simulink model "GCI_Ctrl_PLL_C2000"  (R2024a)
settings: Solver=FixedStepDiscrete  StartTime=0.0  StopTime=8  FixedStep=Sim.ContSampleTime  RelTol=1e-3  EnableMultiTasking=on
values from neighbouring files (symbols this model uses):
  ADPTV = 1.3912    [ModelDD.sldd]
  Ctrl = 0    [ModelDD.sldd]
  EnableMonitors = 0    [ModelDD.sldd]
  FrcPwr = 1    [ModelDD.sldd]
  IdSp = 0.0    [ModelDD.sldd]
  IqSp = 0.0    [ModelDD.sldd]
  ModReq = 1    [ModelDD.sldd]
  PorISel = 0    [ModelDD.sldd]
  PSp = 0.0    [ModelDD.sldd]
  QSp = 0.0    [ModelDD.sldd]
  Sim : value not decoded    [ModelDD.sldd]
  Test = 0    [ModelDD.sldd]
  Var = 650.0    [ModelDD.sldd]
undefined symbols (not defined in the file or in its folder): DiscIntNeverNeededParam, Down, GPTRIP1SEL, GPTRIP2SEL, magnitude, P, TZ1, TZ2, Up
libraries: simulink x38, c2837xDlib x22, c2802xlib x15, slpidlib x9, spsMeanLib x9, spsCurrentMeasurementLib x7, spsThreePhaseVIMeasurementLib x5, spsVoltageMeasurementLib x5, spsTHDLib x4, spsSeriesRLCBranchLib x4, svdutilitieslib x3, c280xlib x3
(part 11 of 11)

== system GCI_Ctrl_PLL_C2000/C2000_SW/CtrlLoop/CurrentController/FeedForward/Subsystem/abc_dqz/Subsystem2 ==
  note: [  al
      |     be  ]
  note: q = -al*sin(wt) + be*cos(wt)
  note: [  cos(wt)   sin(wt)
      |    -sin(wt)    cos(wt)   ]
  note: d = al*cos(wt) + be*sin(wt)
  note: [ d
      |    q ]
  note: *
  note: =
  alpha_beta : Inport
  Ang : Inport  Port=2  PortDimensions=1
  Fcn : Fcn  Expr=u[1]*cos(u[3]) + u[2]*sin(u[3])
  Fcn1 : Fcn  Expr=-u[1]*sin(u[3]) + u[2]*cos(u[3])
  Mux : Mux  Inputs=3
  Mux1 : Mux  Inputs=[2 1]
  Mux2 : Mux  Inputs=[2 1]
  Selector : Selector  InputPortWidth=3  IndexOptions=Index vector (dialog)  Indices=[1 2]  OutputSizes=1
  Selector1 : Selector  InputPortWidth=3  IndexOptions=Index vector (dialog)  Indices=[3]  OutputSizes=1
  dq : Outport  InitialOutput=[0,0]  VectorParamsAs1DForOutWhenUnconnected=off
  wires:
  Selector1/1 -> Mux/3
  Selector/1 -> Mux1/1, Mux2/1
  Mux2/1 -> Fcn1/1
  Mux/1 -> dq/1
  Ang/1 -> Mux1/2, Mux2/2
  Fcn/1 -> Mux/1
  Fcn1/1 -> Mux/2
  Mux1/1 -> Fcn/1
  alpha_beta/1 -> Selector1/1, Selector/1

== system GCI_Ctrl_PLL_C2000/C2000_SW/CtrlLoop/CurrentController/FeedForward/Subsystem/dd_dqz1/LPF ==
  u : Inport
  Alpha : Gain  Gain=(2-w*Ts)/(2+w*Ts)
  Beta : Gain  Gain=(w*Ts)/(2+w*Ts)
  Delay1 : Delay  DelayLength=1  InitialCondition=y_0
  Delay2 : Delay  DelayLength=1
  Sum1 : Sum  Inputs=++|
  Sum2 : Sum  Inputs=|++
  y : Outport  VectorParamsAs1DForOutWhenUnconnected=off
  wires:
  u/1 -> Sum1/1, Delay2/1
  Delay1/1 -> Alpha/1  "y(n-1)"
  Alpha/1 -> Sum2/2
  Delay2/1 -> Sum1/2
  Sum1/1 -> Beta/1
  Beta/1 -> Sum2/1
  Sum2/1 -> Delay1/1, y/1

== system GCI_Ctrl_PLL_C2000/C2000_SW/CtrlLoop/CurrentController/FeedForward/Subsystem/dd_dqz1/LPF1 ==
  u : Inport
  Alpha : Gain  Gain=(2-w*Ts)/(2+w*Ts)
  Beta : Gain  Gain=(w*Ts)/(2+w*Ts)
  Delay1 : Delay  DelayLength=1  InitialCondition=y_0
  Delay2 : Delay  DelayLength=1
  Sum1 : Sum  Inputs=++|
  Sum2 : Sum  Inputs=|++
  y : Outport  VectorParamsAs1DForOutWhenUnconnected=off
  wires:
  Sum2/1 -> y/1, Delay1/1
  Beta/1 -> Sum2/1
  Sum1/1 -> Beta/1
  Delay2/1 -> Sum1/2
  Alpha/1 -> Sum2/2
  Delay1/1 -> Alpha/1  "y(n-1)"
  u/1 -> Delay2/1, Sum1/1

== system GCI_Ctrl_PLL_C2000/C2000_SW/CtrlLoop/CurrentController/FeedForward/Subsystem/dd_dqz1/Subsystem ==
  abc : Inport  PortDimensions=3
  Gain1 : Gain  Gain=single(2/3)  ParamDataTypeStr=single  SaturateOnIntegerOverflow=on  OutDataTypeStr=Inherit: Same as input
  Gain3 : Gain  Gain="single([ 1   -1/2   -1/2; 0   sqrt(3)/2   -sqrt(3)/2; 1/2  1/2  1/2 ] )"  Multiplication=Matrix(K*u) (u vector)  ParamDataTypeStr=single  SaturateOnIntegerOverflow=on  OutDataTypeStr=Inherit: Same as input
  al_be_0 : Outport  VectorParamsAs1DForOutWhenUnconnected=off
  wires:
  abc/1 -> Gain3/1
  Gain3/1 -> Gain1/1
  Gain1/1 -> al_be_0/1  "AlphaBetaZero"

== system GCI_Ctrl_PLL_C2000/C2000_SW/CtrlLoop/CurrentController/FeedForward/Subsystem/dd_dqz1/Subsystem1 ==
  note: =
  note: *
  note: [ d
      |    q ]
  note: d = al*cos(wt) + be*sin(wt)
  note: [  cos(wt)   sin(wt)
      |    -sin(wt)    cos(wt)   ]
  note: q = -al*sin(wt) + be*cos(wt)
  note: [  al
      |     be  ]
  alpha_beta : Inport
  wtNow : Inport  Port=2  PortDimensions=1
  Fcn : Fcn  Expr=u[1]*cos(u[3]) + u[2]*sin(u[3])
  Fcn1 : Fcn  Expr=-u[1]*sin(u[3]) + u[2]*cos(u[3])
  Mux : Mux  Inputs=3
  Mux1 : Mux  Inputs=[2 1]
  Mux2 : Mux  Inputs=[2 1]
  Selector : Selector  InputPortWidth=3  IndexOptions=Index vector (dialog)  Indices=[1 2]  OutputSizes=1
  Selector1 : Selector  InputPortWidth=3  IndexOptions=Index vector (dialog)  Indices=[3]  OutputSizes=1
  dq : Outport  InitialOutput=[0,0]  VectorParamsAs1DForOutWhenUnconnected=off
  wires:
  alpha_beta/1 -> Selector/1, Selector1/1
  Mux1/1 -> Fcn/1
  Fcn1/1 -> Mux/2
  Fcn/1 -> Mux/1
  wtNow/1 -> Mux2/2, Mux1/2
  Mux/1 -> dq/1
  Mux2/1 -> Fcn1/1
  Selector/1 -> Mux2/1, Mux1/1
  Selector1/1 -> Mux/3

== system GCI_Ctrl_PLL_C2000/C2000_SW/CtrlLoop/CurrentController/FeedForward/Subsystem/dd_dqz1/Subsystem2 ==
  note: [  al
      |     be  ]
  note: q = -al*sin(wt) + be*cos(wt)
  note: [  cos(wt)   sin(wt)
      |    -sin(wt)    cos(wt)   ]
  note: d = al*cos(wt) + be*sin(wt)
  note: [ d
      |    q ]
  note: *
  note: =
  alpha_beta : Inport
  wtNow : Inport  Port=2  PortDimensions=1
  Fcn : Fcn  Expr=u[1]*cos(u[3]) + u[2]*sin(u[3])
  Fcn1 : Fcn  Expr=-u[1]*sin(u[3]) + u[2]*cos(u[3])
  Mux : Mux  Inputs=3
  Mux1 : Mux  Inputs=[2 1]
  Mux2 : Mux  Inputs=[2 1]
  Selector : Selector  InputPortWidth=3  IndexOptions=Index vector (dialog)  Indices=[1 2]  OutputSizes=1
  Selector1 : Selector  InputPortWidth=3  IndexOptions=Index vector (dialog)  Indices=[3]  OutputSizes=1
  dq : Outport  InitialOutput=[0,0]  VectorParamsAs1DForOutWhenUnconnected=off
  wires:
  Selector1/1 -> Mux/3
  Selector/1 -> Mux1/1, Mux2/1
  Mux2/1 -> Fcn1/1
  Mux/1 -> dq/1
  Fcn/1 -> Mux/1
  Fcn1/1 -> Mux/2
  Mux1/1 -> Fcn/1
  alpha_beta/1 -> Selector1/1, Selector/1
  wtNow/1 -> Mux2/2, Mux1/2

== system GCI_Ctrl_PLL_C2000/C2000_SW/CtrlLoop/CurrentController/FeedForward/Subsystem/dd_dqz1/Subsystem3 ==
  Vdq_in : Inport
  Vdq_Inverse : Inport  Port=2
  Theta : Inport  Port=3
  Cos : Trigonometry  Operator=cos
  Demux1 : Demux  Outputs=2
  Demux2 : Demux  Outputs=2
  Gain : Gain  Gain=2  ParamDataTypeStr=single
  Ground : Ground
  Mux : Mux  Inputs=3
  Product{,1..3} (4 alike) : Product
  Selector : Selector  InputPortWidth=3  IndexOptions=Index vector (dialog)  Indices=[1 2]  OutputSizes=1
  Selector1 : Selector  InputPortWidth=3  IndexOptions=Index vector (dialog)  Indices=[1 2]  OutputSizes=1
  Sin : Trigonometry
  Sum : Sum  Inputs=|+-
  Sum1 : Sum  Inputs=|++
  Sum2 : Sum  Inputs=|+-
  Sum3 : Sum  Inputs=|+-
  Vdq_out : Outport  VectorParamsAs1DForOutWhenUnconnected=off
  wires:
  Ground/1 -> Mux/3
  Mux/1 -> Vdq_out/1
  Sum3/1 -> Mux/2
  Product3/1 -> Sum3/2
  Sum1/1 -> Sum3/1
  [Vq_Neg] -> Product3/1
  [Cos] -> Product3/2
  Product2/1 -> Sum2/2
  [Vq_Neg] -> Product2/1
  [Sin] -> Product2/2
  Sum2/1 -> Mux/1
  Sum/1 -> Sum2/1
  [Vq_Pos] -> Sum1/1
  Product1/1 -> Sum1/2
  [Vd_Neg] -> Product1/1
  [Sin] -> Product1/2
  [Cos] -> Product/2
  [Vd_Neg] -> Product/1
  Product/1 -> Sum/2
  Cos/1 -> [Cos]
  Sin/1 -> [Sin]
  [Vd_Pos] -> Sum/1
  Demux1/2 -> [Vq_Neg]
  Demux1/1 -> [Vd_Neg]
  Demux2/2 -> [Vq_Pos]
  Demux2/1 -> [Vd_Pos]
  Vdq_Inverse/1 -> Selector1/1
  Selector1/1 -> Demux1/1
  Selector/1 -> Demux2/1
  Vdq_in/1 -> Selector/1
  Gain/1 -> Sin/1, Cos/1
  Theta/1 -> Gain/1

== system GCI_Ctrl_PLL_C2000/C2000_SW/CtrlLoop/CurrentController/FeedForward/Subsystem/dd_dqz1/Subsystem4 ==
  Vdq_in : Inport
  Vdq_Inverse : Inport  Port=2
  Theta : Inport  Port=3
  Cos : Trigonometry  Operator=cos
  Demux1 : Demux  Outputs=2
  Demux2 : Demux  Outputs=2
  Gain : Gain  Gain=2  ParamDataTypeStr=single
  Ground : Ground
  Mux : Mux  Inputs=3
  Product{,1..3} (4 alike) : Product
  Selector : Selector  InputPortWidth=3  IndexOptions=Index vector (dialog)  Indices=[1 2]  OutputSizes=1
  Selector1 : Selector  InputPortWidth=3  IndexOptions=Index vector (dialog)  Indices=[1 2]  OutputSizes=1
  Sin : Trigonometry
  Sum : Sum  Inputs=|+-
  Sum1 : Sum  Inputs=|++
  Sum2 : Sum  Inputs=|+-
  Sum3 : Sum  Inputs=|+-
  Vdq_out : Outport  VectorParamsAs1DForOutWhenUnconnected=off
  wires:
  Theta/1 -> Gain/1
  Gain/1 -> Cos/1, Sin/1
  Vdq_in/1 -> Selector/1
  Selector/1 -> Demux2/1
  Selector1/1 -> Demux1/1
  Vdq_Inverse/1 -> Selector1/1
  Demux2/1 -> [Vd_Pos]
  Demux2/2 -> [Vq_Pos]
  Demux1/1 -> [Vd_Neg]
  Demux1/2 -> [Vq_Neg]
  [Vd_Pos] -> Sum/1
  Sin/1 -> [Sin]
  Cos/1 -> [Cos]
  Product/1 -> Sum/2
  [Vd_Neg] -> Product/1
  [Cos] -> Product/2
  [Sin] -> Product1/2
  [Vd_Neg] -> Product1/1
  Product1/1 -> Sum1/2
  [Vq_Pos] -> Sum1/1
  Sum/1 -> Sum2/1
  Sum2/1 -> Mux/1
  [Sin] -> Product2/2
  [Vq_Neg] -> Product2/1
  Product2/1 -> Sum2/2
  [Cos] -> Product3/2
  [Vq_Neg] -> Product3/1
  Sum1/1 -> Sum3/1
  Product3/1 -> Sum3/2
  Sum3/1 -> Mux/2
  Mux/1 -> Vdq_out/1
  Ground/1 -> Mux/3

== system GCI_Ctrl_PLL_C2000/C2000_SW/CtrlLoop/CurrentController/FeedForward/Subsystem/dd_dqz2/LPF ==
  u : Inport
  Alpha : Gain  Gain=(2-w*Ts)/(2+w*Ts)
  Beta : Gain  Gain=(w*Ts)/(2+w*Ts)
  Delay1 : Delay  DelayLength=1  InitialCondition=y_0
  Delay2 : Delay  DelayLength=1
  Sum1 : Sum  Inputs=++|
  Sum2 : Sum  Inputs=|++
  y : Outport  VectorParamsAs1DForOutWhenUnconnected=off
  wires:
  u/1 -> Sum1/1, Delay2/1
  Delay1/1 -> Alpha/1  "y(n-1)"
  Alpha/1 -> Sum2/2
  Delay2/1 -> Sum1/2
  Sum1/1 -> Beta/1
  Beta/1 -> Sum2/1
  Sum2/1 -> Delay1/1, y/1

== system GCI_Ctrl_PLL_C2000/C2000_SW/CtrlLoop/CurrentController/FeedForward/Subsystem/dd_dqz2/LPF1 ==
  u : Inport
  Alpha : Gain  Gain=(2-w*Ts)/(2+w*Ts)
  Beta : Gain  Gain=(w*Ts)/(2+w*Ts)
  Delay1 : Delay  DelayLength=1  InitialCondition=y_0
  Delay2 : Delay  DelayLength=1
  Sum1 : Sum  Inputs=++|
  Sum2 : Sum  Inputs=|++
  y : Outport  VectorParamsAs1DForOutWhenUnconnected=off
  wires:
  Sum2/1 -> y/1, Delay1/1
  Beta/1 -> Sum2/1
  Sum1/1 -> Beta/1
  Delay2/1 -> Sum1/2
  Alpha/1 -> Sum2/2
  Delay1/1 -> Alpha/1  "y(n-1)"
  u/1 -> Delay2/1, Sum1/1

== system GCI_Ctrl_PLL_C2000/C2000_SW/CtrlLoop/CurrentController/FeedForward/Subsystem/dd_dqz2/Subsystem ==
  abc : Inport  PortDimensions=3
  Gain1 : Gain  Gain=single(2/3)  ParamDataTypeStr=single  SaturateOnIntegerOverflow=on  OutDataTypeStr=Inherit: Same as input
  Gain3 : Gain  Gain="single([ 1   -1/2   -1/2; 0   sqrt(3)/2   -sqrt(3)/2; 1/2  1/2  1/2 ] )"  Multiplication=Matrix(K*u) (u vector)  ParamDataTypeStr=single  SaturateOnIntegerOverflow=on  OutDataTypeStr=Inherit: Same as input
  al_be_0 : Outport  VectorParamsAs1DForOutWhenUnconnected=off
  wires:
  Gain1/1 -> al_be_0/1  "AlphaBetaZero"
  Gain3/1 -> Gain1/1
  abc/1 -> Gain3/1

== system GCI_Ctrl_PLL_C2000/C2000_SW/CtrlLoop/CurrentController/FeedForward/Subsystem/dd_dqz2/Subsystem1 ==
  note: [  al
      |     be  ]
  note: q = -al*sin(wt) + be*cos(wt)
  note: [  cos(wt)   sin(wt)
      |    -sin(wt)    cos(wt)   ]
  note: d = al*cos(wt) + be*sin(wt)
  note: [ d
      |    q ]
  note: *
  note: =
  alpha_beta : Inport
  wtNow : Inport  Port=2  PortDimensions=1
  Fcn : Fcn  Expr=u[1]*cos(u[3]) + u[2]*sin(u[3])
  Fcn1 : Fcn  Expr=-u[1]*sin(u[3]) + u[2]*cos(u[3])
  Mux : Mux  Inputs=3
  Mux1 : Mux  Inputs=[2 1]
  Mux2 : Mux  Inputs=[2 1]
  Selector : Selector  InputPortWidth=3  IndexOptions=Index vector (dialog)  Indices=[1 2]  OutputSizes=1
  Selector1 : Selector  InputPortWidth=3  IndexOptions=Index vector (dialog)  Indices=[3]  OutputSizes=1
  dq : Outport  InitialOutput=[0,0]  VectorParamsAs1DForOutWhenUnconnected=off
  wires:
  Selector1/1 -> Mux/3
  Selector/1 -> Mux1/1, Mux2/1
  Mux2/1 -> Fcn1/1
  Mux/1 -> dq/1  "dq"
  wtNow/1 -> Mux1/2, Mux2/2
  Fcn/1 -> Mux/1
  Fcn1/1 -> Mux/2
  Mux1/1 -> Fcn/1
  alpha_beta/1 -> Selector1/1, Selector/1

== system GCI_Ctrl_PLL_C2000/C2000_SW/CtrlLoop/CurrentController/FeedForward/Subsystem/dd_dqz2/Subsystem2 ==
  note: =
  note: *
  note: [ d
      |    q ]
  note: d = al*cos(wt) + be*sin(wt)
  note: [  cos(wt)   sin(wt)
      |    -sin(wt)    cos(wt)   ]
  note: q = -al*sin(wt) + be*cos(wt)
  note: [  al
      |     be  ]
  alpha_beta : Inport
  wtNow : Inport  Port=2  PortDimensions=1
  Fcn : Fcn  Expr=u[1]*cos(u[3]) + u[2]*sin(u[3])
  Fcn1 : Fcn  Expr=-u[1]*sin(u[3]) + u[2]*cos(u[3])
  Mux : Mux  Inputs=3
  Mux1 : Mux  Inputs=[2 1]
  Mux2 : Mux  Inputs=[2 1]
  Selector : Selector  InputPortWidth=3  IndexOptions=Index vector (dialog)  Indices=[1 2]  OutputSizes=1
  Selector1 : Selector  InputPortWidth=3  IndexOptions=Index vector (dialog)  Indices=[3]  OutputSizes=1
  dq : Outport  InitialOutput=[0,0]  VectorParamsAs1DForOutWhenUnconnected=off
  wires:
  alpha_beta/1 -> Selector/1, Selector1/1
  Mux1/1 -> Fcn/1
  Fcn1/1 -> Mux/2
  Fcn/1 -> Mux/1
  wtNow/1 -> Mux2/2, Mux1/2
  Mux/1 -> dq/1  "dq"
  Mux2/1 -> Fcn1/1
  Selector/1 -> Mux2/1, Mux1/1
  Selector1/1 -> Mux/3

== system GCI_Ctrl_PLL_C2000/C2000_SW/CtrlLoop/CurrentController/FeedForward/Subsystem/dd_dqz2/Subsystem3 ==
  Vdq_in : Inport
  Vdq_Inverse : Inport  Port=2
  Theta : Inport  Port=3
  Cos : Trigonometry  Operator=cos
  Demux1 : Demux  Outputs=2
  Demux2 : Demux  Outputs=2
  Gain : Gain  Gain=2  ParamDataTypeStr=single
  Ground : Ground
  Mux : Mux  Inputs=3
  Product{,1..3} (4 alike) : Product
  Selector : Selector  InputPortWidth=3  IndexOptions=Index vector (dialog)  Indices=[1 2]  OutputSizes=1
  Selector1 : Selector  InputPortWidth=3  IndexOptions=Index vector (dialog)  Indices=[1 2]  OutputSizes=1
  Sin : Trigonometry
  Sum : Sum  Inputs=|+-
  Sum1 : Sum  Inputs=|++
  Sum2 : Sum  Inputs=|+-
  Sum3 : Sum  Inputs=|+-
  Vdq_out : Outport  VectorParamsAs1DForOutWhenUnconnected=off
  wires:
  Theta/1 -> Gain/1
  Gain/1 -> Cos/1, Sin/1
  Vdq_in/1 -> Selector/1
  Selector/1 -> Demux2/1
  Selector1/1 -> Demux1/1
  Vdq_Inverse/1 -> Selector1/1
  Demux2/1 -> [Vd_Pos]
  Demux2/2 -> [Vq_Pos]
  Demux1/1 -> [Vd_Neg]
  Demux1/2 -> [Vq_Neg]
  [Vd_Pos] -> Sum/1
  Sin/1 -> [Sin]
  Cos/1 -> [Cos]
  Product/1 -> Sum/2
  [Vd_Neg] -> Product/1
  [Cos] -> Product/2
  [Sin] -> Product1/2
  [Vd_Neg] -> Product1/1
  Product1/1 -> Sum1/2
  [Vq_Pos] -> Sum1/1
  Sum/1 -> Sum2/1
  Sum2/1 -> Mux/1
  [Sin] -> Product2/2
  [Vq_Neg] -> Product2/1
  Product2/1 -> Sum2/2
  [Cos] -> Product3/2
  [Vq_Neg] -> Product3/1
  Sum1/1 -> Sum3/1
  Product3/1 -> Sum3/2
  Sum3/1 -> Mux/2
  Mux/1 -> Vdq_out/1
  Ground/1 -> Mux/3

== system GCI_Ctrl_PLL_C2000/C2000_SW/CtrlLoop/CurrentController/FeedForward/Subsystem/dd_dqz2/Subsystem4 ==
  Vdq_in : Inport
  Vdq_Inverse : Inport  Port=2
  Theta : Inport  Port=3
  Cos : Trigonometry  Operator=cos
  Demux1 : Demux  Outputs=2
  Demux2 : Demux  Outputs=2
  Gain : Gain  Gain=2  ParamDataTypeStr=single
  Ground : Ground
  Mux : Mux  Inputs=3
  Product{,1..3} (4 alike) : Product
  Selector : Selector  InputPortWidth=3  IndexOptions=Index vector (dialog)  Indices=[1 2]  OutputSizes=1
  Selector1 : Selector  InputPortWidth=3  IndexOptions=Index vector (dialog)  Indices=[1 2]  OutputSizes=1
  Sin : Trigonometry
  Sum : Sum  Inputs=|+-
  Sum1 : Sum  Inputs=|++
  Sum2 : Sum  Inputs=|+-
  Sum3 : Sum  Inputs=|+-
  Vdq_out : Outport  VectorParamsAs1DForOutWhenUnconnected=off
  wires:
  Ground/1 -> Mux/3
  Mux/1 -> Vdq_out/1
  Sum3/1 -> Mux/2
  Product3/1 -> Sum3/2
  Sum1/1 -> Sum3/1
  [Vq_Neg] -> Product3/1
  [Cos] -> Product3/2
  Product2/1 -> Sum2/2
  [Vq_Neg] -> Product2/1
  [Sin] -> Product2/2
  Sum2/1 -> Mux/1
  Sum/1 -> Sum2/1
  [Vq_Pos] -> Sum1/1
  Product1/1 -> Sum1/2
  [Vd_Neg] -> Product1/1
  [Sin] -> Product1/2
  [Cos] -> Product/2
  [Vd_Neg] -> Product/1
  Product/1 -> Sum/2
  Cos/1 -> [Cos]
  Sin/1 -> [Sin]
  [Vd_Pos] -> Sum/1
  Demux1/2 -> [Vq_Neg]
  Demux1/1 -> [Vd_Neg]
  Demux2/2 -> [Vq_Pos]
  Demux2/1 -> [Vd_Pos]
  Vdq_Inverse/1 -> Selector1/1
  Selector1/1 -> Demux1/1
  Selector/1 -> Demux2/1
  Vdq_in/1 -> Selector/1
  Gain/1 -> Sin/1, Cos/1
  Theta/1 -> Gain/1

== system GCI_Ctrl_PLL_C2000/C2000_SW/CtrlLoop/PLL_Vref/abc2dqzFilt/Single_SOGI/Subsystem1/SOGI_QSG ==
  U : Inport
  wo : Inport  Port=2
  Delay : Delay  DelayLength=1
  Discrete-Time Integrator : DiscreteIntegrator  gainval=single(1)  InitialCondition=single(0)  SampleTime=-1  ICPrevOutput=DiscIntNeverNeededParam  ICPrevScaledInput=DiscIntNeverNeededParam
  Discrete-Time Integrator1 : DiscreteIntegrator  gainval=single(1)  InitialCondition=single(0)  SampleTime=-1  ICPrevOutput=DiscIntNeverNeededParam  ICPrevScaledInput=DiscIntNeverNeededParam
  Gain : Gain  Gain=Var.SogiK  ParamDataTypeStr=single
  Product : Product
  Product1 : Product
  Saturation : Saturate  UpperLimit=single(2*pi*65)  LowerLimit=single(2*pi*30)
  Sum : Sum  Inputs=-+|
  Sum1 : Sum  Inputs=|+-
  Y : Outport  VectorParamsAs1DForOutWhenUnconnected=off
  qY : Outport  Port=2  VectorParamsAs1DForOutWhenUnconnected=off
  wires:
  Saturation/1 -> Product1/1, Product/2
  Delay/1 -> Saturation/1
  Discrete-Time Integrator1/1 -> Sum1/2, qY/1
  Discrete-Time Integrator/1 -> Sum/1, Y/1, Product1/2
  Sum/1 -> Gain/1
  Gain/1 -> Sum1/1
  Product1/1 -> Discrete-Time Integrator1/1
  U/1 -> Sum/2
  Product/1 -> Discrete-Time Integrator/1
  wo/1 -> Delay/1
  Sum1/1 -> Product/1

== system GCI_Ctrl_PLL_C2000/C2000_SW/CtrlLoop/PLL_Vref/abc2dqzFilt/dd_dqz_SOGI/Subsystem5/SOGI_QSG ==
  U : Inport
  wo : Inport  Port=2
  Delay : Delay  DelayLength=1
  Discrete-Time Integrator : DiscreteIntegrator  gainval=single(1)  InitialCondition=single(0)  SampleTime=-1  ICPrevOutput=DiscIntNeverNeededParam  ICPrevScaledInput=DiscIntNeverNeededParam
  Discrete-Time Integrator1 : DiscreteIntegrator  gainval=single(1)  InitialCondition=single(0)  SampleTime=-1  ICPrevOutput=DiscIntNeverNeededParam  ICPrevScaledInput=DiscIntNeverNeededParam
  Gain : Gain  Gain=Var.SogiK  ParamDataTypeStr=single
  Product : Product
  Product1 : Product
  Saturation : Saturate  UpperLimit=single(2*pi*55)  LowerLimit=single(2*pi*45)
  Sum : Sum  Inputs=-+|
  Sum1 : Sum  Inputs=|+-
  Y : Outport  VectorParamsAs1DForOutWhenUnconnected=off
  qY : Outport  Port=2  VectorParamsAs1DForOutWhenUnconnected=off
  wires:
  Sum1/1 -> Product/1
  wo/1 -> Delay/1
  Product/1 -> Discrete-Time Integrator/1
  U/1 -> Sum/2
  Product1/1 -> Discrete-Time Integrator1/1
  Gain/1 -> Sum1/1
  Sum/1 -> Gain/1
  Discrete-Time Integrator/1 -> Product1/2, Y/1, Sum/1
  Discrete-Time Integrator1/1 -> qY/1, Sum1/2
  Delay/1 -> Saturation/1
  Saturation/1 -> Product/2, Product1/1

== system GCI_Ctrl_PLL_C2000/C2000_SW/CtrlLoop/PLL_Vref/abc2dqzFilt/dd_dqz_SOGI/dqz_SOGI/Subsystem ==
  abc : Inport  PortDimensions=3
  Gain1 : Gain  Gain=single(2/3)  ParamDataTypeStr=single  SaturateOnIntegerOverflow=on  OutDataTypeStr=Inherit: Same as input
  Gain3 : Gain  Gain="single([ 1   -1/2   -1/2; 0   sqrt(3)/2   -sqrt(3)/2; 1/2  1/2  1/2 ] )"  Multiplication=Matrix(K*u) (u vector)  ParamDataTypeStr=single  SaturateOnIntegerOverflow=on  OutDataTypeStr=Inherit: Same as input
  al_be_0 : Outport  VectorParamsAs1DForOutWhenUnconnected=off
  wires:
  Gain1/1 -> al_be_0/1
  Gain3/1 -> Gain1/1
  abc/1 -> Gain3/1

== system GCI_Ctrl_PLL_C2000/C2000_SW/CtrlLoop/PLL_Vref/abc2dqzFilt/dd_dqz_SOGI/dqz_SOGI/Subsystem1 ==
  AlphBeta : Inport
  w : Inport  Port=2
  Demux : Demux  Outputs=2
  Demux1 : Demux  Outputs=2
  Gain : Gain  Gain=single(1/3)  ParamDataTypeStr=single
  Gain1 : Gain  Gain=single(1/3)  ParamDataTypeStr=single
  Ground : Ground
  Mux : Mux  Inputs=3
  SOGI_QSG : Subsystem
  Selector1 : Selector  InputPortWidth=3  IndexOptions=Index vector (dialog)  Indices=[1 2]  OutputSizes=1
  Sum : Sum  Inputs=|+-
  Sum1 : Sum  Inputs=|++
  AlphBetaCor : Outport  VectorParamsAs1DForOutWhenUnconnected=off
  wires:
  AlphBeta/1 -> Selector1/1
  SOGI_QSG/2(qY) -> Demux1/1
  Selector1/1 -> SOGI_QSG/1(U)
  Demux/2 -> Sum1/1
  Demux/1 -> Sum/1
  Demux1/2 -> Sum/2
  Demux1/1 -> Sum1/2
  Sum/1 -> Gain/1
  Sum1/1 -> Gain1/1
  Ground/1 -> Mux/3
  Mux/1 -> AlphBetaCor/1
  w/1 -> SOGI_QSG/2(wo)
  SOGI_QSG/1(Y) -> Demux/1
  Gain/1 -> Mux/1
  Gain1/1 -> Mux/2

== system GCI_Ctrl_PLL_C2000/C2000_SW/CtrlLoop/PLL_Vref/abc2dqzFilt/dd_dqz_SOGI/dqz_SOGI/Subsystem2 ==
  note: =
  note: *
  note: [ d
      |    q ]
  note: d = al*cos(wt) + be*sin(wt)
  note: [  cos(wt)   sin(wt)
      |    -sin(wt)    cos(wt)   ]
  note: q = -al*sin(wt) + be*cos(wt)
  note: [  al
      |     be  ]
  alpha_beta : Inport
  Ang : Inport  Port=2  PortDimensions=1
  Fcn : Fcn  Expr=u[1]*cos(u[3]) + u[2]*sin(u[3])
  Fcn1 : Fcn  Expr=-u[1]*sin(u[3]) + u[2]*cos(u[3])
  Mux : Mux  Inputs=3
  Mux1 : Mux  Inputs=[2 1]
  Mux2 : Mux  Inputs=[2 1]
  Selector : Selector  InputPortWidth=3  IndexOptions=Index vector (dialog)  Indices=[1 2]  OutputSizes=1
  Selector1 : Selector  InputPortWidth=3  IndexOptions=Index vector (dialog)  Indices=[3]  OutputSizes=1
  dq : Outport  InitialOutput=[0,0]  VectorParamsAs1DForOutWhenUnconnected=off
  wires:
  alpha_beta/1 -> Selector/1, Selector1/1
  Mux1/1 -> Fcn/1
  Fcn1/1 -> Mux/2
  Fcn/1 -> Mux/1
  Ang/1 -> Mux2/2, Mux1/2
  Mux/1 -> dq/1
  Mux2/1 -> Fcn1/1
  Selector/1 -> Mux2/1, Mux1/1
  Selector1/1 -> Mux/3

== system GCI_Ctrl_PLL_C2000/C2000_SW/CtrlLoop/PLL_Vref/abc2dqzFilt/dd_dqz_SOGI/dqz_SOGI/Subsystem3 ==
  note: [  al
      |     be  ]
  note: q = -al*sin(wt) + be*cos(wt)
  note: [  cos(wt)   sin(wt)
      |    -sin(wt)    cos(wt)   ]
  note: d = al*cos(wt) + be*sin(wt)
  note: [ d
      |    q ]
  note: *
  note: =
  alpha_beta : Inport
  Ang : Inport  Port=2  PortDimensions=1
  Fcn : Fcn  Expr=u[1]*cos(u[3]) + u[2]*sin(u[3])
  Fcn1 : Fcn  Expr=-u[1]*sin(u[3]) + u[2]*cos(u[3])
  Mux : Mux  Inputs=3
  Mux1 : Mux  Inputs=[2 1]
  Mux2 : Mux  Inputs=[2 1]
  Selector : Selector  InputPortWidth=3  IndexOptions=Index vector (dialog)  Indices=[1 2]  OutputSizes=1
  Selector1 : Selector  InputPortWidth=3  IndexOptions=Index vector (dialog)  Indices=[3]  OutputSizes=1
  dq : Outport  InitialOutput=[0,0]  VectorParamsAs1DForOutWhenUnconnected=off
  wires:
  Selector1/1 -> Mux/3
  Selector/1 -> Mux1/1, Mux2/1
  Mux2/1 -> Fcn1/1
  Mux/1 -> dq/1
  Ang/1 -> Mux1/2, Mux2/2
  Fcn/1 -> Mux/1
  Fcn1/1 -> Mux/2
  Mux1/1 -> Fcn/1
  alpha_beta/1 -> Selector1/1, Selector/1

== system GCI_Ctrl_PLL_C2000/C2000_SW/CtrlLoop/PLL_Vref/abc2dqzFilt/dqz_1P_SOGI_Disc/SOGI/SOGI_QSG ==
  U : Inport
  wo : Inport  Port=2
  Delay4 : Delay  DelayLength=1
  Subsystem : Subsystem
  Subsystem1 : Subsystem
  Terminator : Terminator
  Y : Outport  VectorParamsAs1DForOutWhenUnconnected=off
  qY : Outport  Port=2  VectorParamsAs1DForOutWhenUnconnected=off
  wires:
  Subsystem/4(b2) -> Terminator/1
  Subsystem/3(a2) -> Subsystem1/5(a2)
  Subsystem/2(a1) -> Subsystem1/4(a1)
  Subsystem/1(b0) -> Subsystem1/3(b0)
  Subsystem1/2(qY) -> qY/1
  Subsystem1/1(Y) -> Y/1
  U/1 -> Subsystem1/1(U)
  wo/1 -> Delay4/1
  Delay4/1 -> Subsystem/1(w), Subsystem1/2(w)

== system GCI_Ctrl_PLL_C2000/C2000_SW/CtrlLoop/PLL_Vref/abc2dqzFilt/dqz_DSOGI/SOGI/SOGI_QSG ==
  U : Inport
  wo : Inport  Port=2
  Delay : Delay  DelayLength=1
  Discrete-Time Integrator : DiscreteIntegrator  gainval=single(1)  InitialCondition=single(0)  SampleTime=-1  ICPrevOutput=DiscIntNeverNeededParam  ICPrevScaledInput=DiscIntNeverNeededParam
  Discrete-Time Integrator1 : DiscreteIntegrator  gainval=single(1)  InitialCondition=single(0)  SampleTime=-1  ICPrevOutput=DiscIntNeverNeededParam  ICPrevScaledInput=DiscIntNeverNeededParam
  Gain : Gain  Gain=Var.SogiK  ParamDataTypeStr=single
  Product : Product
  Product1 : Product
  Sum : Sum  Inputs=-+|
  Sum1 : Sum  Inputs=|+-
  Y : Outport  VectorParamsAs1DForOutWhenUnconnected=off
  qY : Outport  Port=2  VectorParamsAs1DForOutWhenUnconnected=off
  wires:
  Delay/1 -> Product1/1, Product/2
  Discrete-Time Integrator1/1 -> Sum1/2, qY/1
  Discrete-Time Integrator/1 -> Sum/1, Y/1, Product1/2
  Sum/1 -> Gain/1
  Gain/1 -> Sum1/1
  Product1/1 -> Discrete-Time Integrator1/1
  U/1 -> Sum/2
  Product/1 -> Discrete-Time Integrator/1
  wo/1 -> Delay/1
  Sum1/1 -> Product/1

== system GCI_Ctrl_PLL_C2000/C2000_SW/CtrlLoop/PLL_Vref/abc2dqzFilt/dqz_SOGI/SOGI/SOGI_QSG ==
  U : Inport
  wo : Inport  Port=2
  Abs : Abs  SaturateOnIntegerOverflow=off
  Compare To Constant : simulink/Logic and Bit Operations/Compare To Constant  relop=>=  const=2000  OutDataTypeStr=boolean
  Constant : Constant  Value=eps  OutDataTypeStr=single
  Delay : Delay  DelayLength=1
  Discrete-Time Integrator : DiscreteIntegrator  gainval=single(1)  ExternalReset=rising  InitialCondition=single(0)  SampleTime=-1  ICPrevOutput=DiscIntNeverNeededParam  ICPrevScaledInput=DiscIntNeverNeededParam
  Discrete-Time Integrator1 : DiscreteIntegrator  gainval=single(1)  ExternalReset=rising  InitialCondition=single(0)  SampleTime=-1  ICPrevOutput=DiscIntNeverNeededParam  ICPrevScaledInput=DiscIntNeverNeededParam
  Gain : Gain  Gain=Var.SogiK  ParamDataTypeStr=single
  Max : MinMax  Function=max  Inputs=2
  Product : Product
  Product1 : Product
  Product2 : Product
  Saturation1 : Saturate  Commented=on  UpperLimit=single(2*pi*65)  LowerLimit=single(2*pi*30)
  Sign : Signum
  Sqrt : Sqrt
  Square : Math  Operator=square
  Sum : Sum  Inputs=-+|
  Sum of Elements : Sum  Inputs=+
  Sum1 : Sum  Inputs=|+-
  Unit Delay : UnitDelay  SampleTime=-1  HasFrameUpgradeWarning=on
  Y : Outport  VectorParamsAs1DForOutWhenUnconnected=off
  qY : Outport  Port=2  VectorParamsAs1DForOutWhenUnconnected=off
  wires:
  Sum1/1 -> Product/1
  wo/1 -> Delay/1
  Product/1 -> Discrete-Time Integrator/1
  U/1 -> Sum/2
  Product1/1 -> Discrete-Time Integrator1/1
  Gain/1 -> Sum1/1
  Sum/1 -> Gain/1
  Discrete-Time Integrator/1 -> Sum/1, Square/1, Y/1, Product1/2
  Discrete-Time Integrator1/1 -> Sum1/2, qY/1
  Product2/1 -> Product/2, Product1/1
  Square/1 -> Sum of Elements/1
  Sum of Elements/1 -> Sqrt/1
  Sqrt/1 -> Compare To Constant/1
  Compare To Constant/1 -> Unit Delay/1
  Unit Delay/1 -> Discrete-Time Integrator1/2, Discrete-Time Integrator/2
  Delay/1 -> Sign/1, Abs/1
  Abs/1 -> Max/1
  Constant/1 -> Max/2
  Max/1 -> Product2/1
  Sign/1 -> Product2/2

== system GCI_Ctrl_PLL_C2000/C2000_SW/CtrlLoop/PLL_Vref/abc2dqzFilt/dqz_SOGI_ConstW/Subsystem1/SOGI_QSG ==
  U : Inport
  wo : Inport  Port=2
  Constant : Constant  Value=2*pi*Var.Grid_Frq
  Discrete-Time Integrator : DiscreteIntegrator  gainval=single(1)  InitialCondition=single(0)  SampleTime=-1  ICPrevOutput=DiscIntNeverNeededParam  ICPrevScaledInput=DiscIntNeverNeededParam
  Discrete-Time Integrator1 : DiscreteIntegrator  gainval=single(1)  InitialCondition=single(0)  SampleTime=-1  ICPrevOutput=DiscIntNeverNeededParam  ICPrevScaledInput=DiscIntNeverNeededParam
  Gain : Gain  Gain=Var.SogiK  ParamDataTypeStr=single
  Product : Product
  Product1 : Product
  Sum : Sum  Inputs=-+|
  Sum1 : Sum  Inputs=|+-
  Terminator : Terminator
  Y : Outport  VectorParamsAs1DForOutWhenUnconnected=off
  qY : Outport  Port=2  VectorParamsAs1DForOutWhenUnconnected=off
  wires:
  Constant/1 -> Product1/1, Product/2
  Discrete-Time Integrator1/1 -> Sum1/2, qY/1
  Discrete-Time Integrator/1 -> Sum/1, Y/1, Product1/2
  Sum/1 -> Gain/1
  Gain/1 -> Sum1/1
  Product1/1 -> Discrete-Time Integrator1/1
  U/1 -> Sum/2
  Product/1 -> Discrete-Time Integrator/1
  Sum1/1 -> Product/1
  wo/1 -> Terminator/1

== system GCI_Ctrl_PLL_C2000/C2000_SW/CtrlLoop/PLL_Vref/abc2dqzFilt/dqz_SOGI_Disc/SOGI/SOGI_QSG ==
  U : Inport
  wo : Inport  Port=2
  Delay4 : Delay  DelayLength=1
  Subsystem : Subsystem
  Subsystem1 : Subsystem
  Terminator : Terminator
  Y : Outport  VectorParamsAs1DForOutWhenUnconnected=off
  qY : Outport  Port=2  VectorParamsAs1DForOutWhenUnconnected=off
  wires:
  wo/1 -> Delay4/1
  Delay4/1 -> Subsystem1/2(w), Subsystem/1(w)
  U/1 -> Subsystem1/1(U)
  Subsystem1/1(Y) -> Y/1
  Subsystem1/2(qY) -> qY/1
  Subsystem/1(b0) -> Subsystem1/3(b0)
  Subsystem/2(a1) -> Subsystem1/4(a1)
  Subsystem/3(a2) -> Subsystem1/5(a2)
  Subsystem/4(b2) -> Terminator/1

== system GCI_Ctrl_PLL_C2000/C2000_SW/CtrlLoop/PLL_Vref/abc2dqzFilt/dd_dqz_SOGI/dqz_SOGI/Subsystem1/SOGI_QSG ==
  U : Inport
  wo : Inport  Port=2
  Delay : Delay  DelayLength=1
  Discrete-Time Integrator : DiscreteIntegrator  gainval=single(1)  InitialCondition=single(0)  SampleTime=-1  ICPrevOutput=DiscIntNeverNeededParam  ICPrevScaledInput=DiscIntNeverNeededParam
  Discrete-Time Integrator1 : DiscreteIntegrator  gainval=single(1)  InitialCondition=single(0)  SampleTime=-1  ICPrevOutput=DiscIntNeverNeededParam  ICPrevScaledInput=DiscIntNeverNeededParam
  Gain : Gain  Gain=Var.SogiK  ParamDataTypeStr=single
  Product : Product
  Product1 : Product
  Saturation : Saturate  UpperLimit=single(2*pi*55)  LowerLimit=single(2*pi*45)
  Sum : Sum  Inputs=-+|
  Sum1 : Sum  Inputs=|+-
  Y : Outport  VectorParamsAs1DForOutWhenUnconnected=off
  qY : Outport  Port=2  VectorParamsAs1DForOutWhenUnconnected=off
  wires:
  Sum1/1 -> Product/1
  wo/1 -> Delay/1
  Product/1 -> Discrete-Time Integrator/1
  U/1 -> Sum/2
  Product1/1 -> Discrete-Time Integrator1/1
  Gain/1 -> Sum1/1
  Sum/1 -> Gain/1
  Discrete-Time Integrator/1 -> Product1/2, Y/1, Sum/1
  Discrete-Time Integrator1/1 -> qY/1, Sum1/2
  Delay/1 -> Saturation/1
  Saturation/1 -> Product/2, Product1/1

== system GCI_Ctrl_PLL_C2000/C2000_SW/CtrlLoop/PLL_Vref/abc2dqzFilt/dqz_1P_SOGI_Disc/SOGI/SOGI_QSG/Subsystem ==
  w : Inport
  Constant : Constant  Value=single(4)
  Constant2 : Constant  Value=single(4)
  Constant3 : Constant  Value=single(4)
  Divide : Product  Inputs=*/
  Divide1 : Product  Inputs=*/
  Divide2 : Product  Inputs=*/
  Gain1 : Gain  Gain=(2*Var.SogiK)  ParamDataTypeStr=single
  Gain2 : Gain  Gain=(1/Var.PWM_Freq)  ParamDataTypeStr=single
  Gain3 : Gain  Gain=single(-1)  ParamDataTypeStr=single
  Gain4 : Gain  Gain=(1/Var.PWM_Freq)  ParamDataTypeStr=single
  Gain5 : Gain  Gain=single(2)  ParamDataTypeStr=single
  Square : Math  Operator=square  SignedPower=on
  Sum2 : Sum  Inputs=+++
  Sum4 : Sum  Inputs=+-|
  Sum5 : Sum  Inputs=+--
  b0 : Outport  VectorParamsAs1DForOutWhenUnconnected=off
  a1 : Outport  Port=2  VectorParamsAs1DForOutWhenUnconnected=off
  a2 : Outport  Port=3  VectorParamsAs1DForOutWhenUnconnected=off
  b2 : Outport  Port=4  VectorParamsAs1DForOutWhenUnconnected=off
  wires:
  Gain2/1 -> Square/1  "w*Ts"
  Gain1/1 -> Gain4/1  "2*k*w"
  Gain3/1 -> b2/1  "b2"
  Divide2/1 -> a2/1  "a2"
  Divide1/1 -> a1/1  "a1"
  Constant3/1 -> Sum5/3
  Constant2/1 -> Sum4/1
  [y] -> Sum4/2
  [y] -> Sum2/2
  Square/1 -> [y]  "y = (w*Ts)^2"
  [x] -> Sum5/1
  w/1 -> Gain1/1, Gain2/1
  Gain5/1 -> Divide1/1  "2(4-y)"
  [y] -> Sum5/2
  Divide/1 -> Gain3/1, b0/1  "b0"
  Constant/1 -> Sum2/3
  Gain4/1 -> [x]  "x = 2*k*w*Ts"
  Sum2/1 -> Divide/2, Divide1/2, Divide2/2  "x+y+4"
  Sum5/1 -> Divide2/1  "x-y-4"
  [x] -> Sum2/1, Divide/1
  Sum4/1 -> Gain5/1

== system GCI_Ctrl_PLL_C2000/C2000_SW/CtrlLoop/PLL_Vref/abc2dqzFilt/dqz_1P_SOGI_Disc/SOGI/SOGI_QSG/Subsystem1 ==
  U : Inport
  w : Inport  Port=2
  b0 : Inport  Port=3
  a1 : Inport  Port=4
  a2 : Inport  Port=5
  Gain : Gain  Gain=2*(1/Var.PWM_Freq)  ParamDataTypeStr=single
  Product{,1..3} (4 alike) : Product
  Sum : Sum  Inputs=|++
  Sum1 : Sum  Inputs=|+-
  Sum3 : Sum  Inputs=++|
  Unit Delay : UnitDelay  SampleTime=-1  HasFrameUpgradeWarning=on
  Unit Delay1 : UnitDelay  SampleTime=-1  HasFrameUpgradeWarning=on
  Y : Outport  VectorParamsAs1DForOutWhenUnconnected=off
  qY : Outport  Port=2  VectorParamsAs1DForOutWhenUnconnected=off
  wires:
  Gain/1 -> Product/1
  a1/1 -> Product1/1
  Product2/1 -> Sum3/2
  Product/1 -> qY/1
  w/1 -> Gain/1
  U/1 -> Product3/1
  Sum3/1 -> Sum/2
  a2/1 -> Product2/2
  Sum1/1 -> Y/1
  Unit Delay1/1 -> Product2/1, Sum1/2
  Product1/1 -> Sum3/1
  Unit Delay/1 -> Product1/2, Unit Delay1/1, Product/2
  Product3/1 -> Sum/1
  b0/1 -> Product3/2
  Sum/1 -> Unit Delay/1, Sum1/1

== system GCI_Ctrl_PLL_C2000/C2000_SW/CtrlLoop/PLL_Vref/abc2dqzFilt/dqz_SOGI_Disc/SOGI/SOGI_QSG/Subsystem ==
  w : Inport
  Constant : Constant  Value=single(4)
  Constant2 : Constant  Value=single(4)
  Constant3 : Constant  Value=single(4)
  Divide : Product  Inputs=*/
  Divide1 : Product  Inputs=*/
  Divide2 : Product  Inputs=*/
  Gain1 : Gain  Gain=(2*Var.SogiK)  ParamDataTypeStr=single
  Gain2 : Gain  Gain=(1/Var.PWM_Freq)  ParamDataTypeStr=single
  Gain3 : Gain  Gain=single(-1)  ParamDataTypeStr=single
  Gain4 : Gain  Gain=(1/Var.PWM_Freq)  ParamDataTypeStr=single
  Gain5 : Gain  Gain=single(2)  ParamDataTypeStr=single
  Square : Math  Operator=square  SignedPower=on
  Sum2 : Sum  Inputs=+++
  Sum4 : Sum  Inputs=+-|
  Sum5 : Sum  Inputs=+--
  b0 : Outport  VectorParamsAs1DForOutWhenUnconnected=off
  a1 : Outport  Port=2  VectorParamsAs1DForOutWhenUnconnected=off
  a2 : Outport  Port=3  VectorParamsAs1DForOutWhenUnconnected=off
  b2 : Outport  Port=4  VectorParamsAs1DForOutWhenUnconnected=off
  wires:
  Sum4/1 -> Gain5/1
  [x] -> Divide/1, Sum2/1
  Sum5/1 -> Divide2/1  "xMinusyMinusFour"
  Sum2/1 -> Divide2/2, Divide1/2, Divide/2  "xPlusyPlusFour"
  Gain4/1 -> [x]  "TwokwTs"
  Constant/1 -> Sum2/3
  Divide/1 -> b0/1, Gain3/1  "b0"
  [y] -> Sum5/2
  Gain5/1 -> Divide1/1  "Two_FourMinusy"
  w/1 -> Gain2/1, Gain1/1
  [x] -> Sum5/1
  Square/1 -> [y]  "wTs_sq"
  [y] -> Sum2/2
  [y] -> Sum4/2
  Constant2/1 -> Sum4/1
  Constant3/1 -> Sum5/3
  Divide1/1 -> a1/1  "a1"
  Divide2/1 -> a2/1  "a2"
  Gain3/1 -> b2/1  "b2"
  Gain1/1 -> Gain4/1  "Twokw"
  Gain2/1 -> Square/1  "wTs"

== system GCI_Ctrl_PLL_C2000/C2000_SW/CtrlLoop/PLL_Vref/abc2dqzFilt/dqz_SOGI_Disc/SOGI/SOGI_QSG/Subsystem1 ==
  U : Inport
  w : Inport  Port=2
  b0 : Inport  Port=3
  a1 : Inport  Port=4
  a2 : Inport  Port=5
  Gain : Gain  Gain=2*(1/Var.PWM_Freq)  ParamDataTypeStr=single
  Product{,1..3} (4 alike) : Product
  Sum : Sum  Inputs=|++
  Sum1 : Sum  Inputs=|+-
  Sum3 : Sum  Inputs=++|
  Unit Delay : UnitDelay  SampleTime=-1  HasFrameUpgradeWarning=on
  Unit Delay1 : UnitDelay  SampleTime=-1  HasFrameUpgradeWarning=on
  Y : Outport  VectorParamsAs1DForOutWhenUnconnected=off
  qY : Outport  Port=2  VectorParamsAs1DForOutWhenUnconnected=off
  wires:
  Sum/1 -> Sum1/1, Unit Delay/1
  b0/1 -> Product3/2
  Product3/1 -> Sum/1
  Unit Delay/1 -> Product/2, Unit Delay1/1, Product1/2
  Product1/1 -> Sum3/1
  Unit Delay1/1 -> Sum1/2, Product2/1
  Sum1/1 -> Y/1  "VgAlphaQBetaPll"
  a2/1 -> Product2/2
  Sum3/1 -> Sum/2
  U/1 -> Product3/1
  w/1 -> Gain/1
  Product/1 -> qY/1  "VgQAlphaBetaPll"
  Product2/1 -> Sum3/2
  a1/1 -> Product1/1
  Gain/1 -> Product/1

== stateflow chart GCI_Ctrl_PLL_C2000/C2000_SW/SysSts/States ==
  state States
    state Standby
      SafeState = 1;
      ControllerEn = 0;
      PllEn = 1;
    state Power
      SafeState = 0;
      ControllerEn = 1;
      PllEn = 1;
    state Failure
      SafeState = 1;
      ControllerEn = 0;
      PllEn = 0;
    (default) -> Standby
    Standby -> Power [order 1] : [((MdReq == 1 ...
        | & SysStsSynch == 1 ...
        | & HvdcUAct > Var.States_HvdcUActMin ...
        | & HvacUMinAct > Var.States_HvacUActMin ) ...
        | | FrcPwr ==  1) && after(Var.States_StdbyToPwrTime, msec)] ...
    Standby -> Failure [order 2] : [SysStsFail == 1 ...
        | & EnaMon == 1]
    Power -> Failure [order 2] : [SysStsFail == 1 ...
        | & EnaMon == 1]
    Power -> Standby [order 1] : [(MdReq == 0 ...
        | | SysStsSynch == 0 ...
        | | HvdcUAct < Var.States_HvdcUActMin ...
        | | HvacUMinAct < Var.States_HvacUActMin )...
        | &  FrcPwr == 0]
    Failure -> Standby : [SysStsFail == 0 ...
        | | EnaMon == 0]
  data: StatesMode output Enum: StatesModeType; FrcPwr input; MdReq input; HvdcUAct input; SafeState output boolean; HvacUMinAct input; Var parameter; SysStsFail input; ControllerEn output boolean; SysStsSynch input; PllEn output boolean; EnaMon input
